simulink model "compDigital2"  (R2018a)
settings: Solver=VariableStepAuto  StartTime=0.0  StopTime=10.0  RelTol=1e-3
values from neighbouring files (symbols this model uses):
  Ts = 1/fs    (= 2e-05)    [transferencias_digitales.m]
undefined symbols (not defined in the file or in its folder): CtotalZ, Gtotalz, intZ
libraries: simulink x1
settings Model: Creator=Ignacio  LastModifiedBy=Ignacio

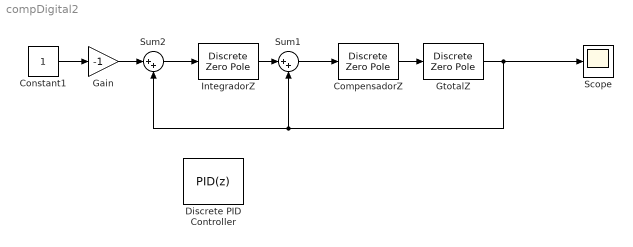
== system compDigital2 ==
  CompensadorZ : DiscreteZeroPole  Zeros=CtotalZ.Z{1,1}  Poles=CtotalZ.P{1,1}  Gain=CtotalZ.K  SampleTime=Ts
  Constant1 : Constant
  Discrete PID Controller : simulink/Continuous/PID Controller  Controller=PID  TimeDomain=Discrete-time  SampleTime=-1  IntegratorMethod=Forward Euler  FilterMethod=Forward Euler  Form=Parallel  UseFilter=on  ControllerParametersSource=internal  P=1  I=1  D=0  N=100  InitialConditionSource=internal  InitialConditionForIntegrator=0  InitialConditionForFilter=0  ExternalReset=none  LimitOutput=off  UpperSaturationLimit=inf  LowerSaturationLimit=-inf  LinearizeAsGain=off  AntiWindupMode=none  Kb=1  TrackingMode=off  Kt=1  PParamMin=[]  PParamMax=[]  IParamMin=[]  IParamMax=[]  DParamMin=[]  DParamMax=[]  NParamMin=[]  NParamMax=[]  KbParamMin=[]  KbParamMax=[]  KtParamMin=[]  KtParamMax=[]  POutMin=[]  POutMax=[]  IOutMin=[]  IOutMax=[]  DOutMin=[]  DOutMax=[]  NOutMin=[]  NOutMax=[]  KbOutMin=[]  KbOutMax=[]  KtOutMin=[]  KtOutMax=[]  IntegratorOutMin=[]  IntegratorOutMax=[]  FilterOutMin=[]  FilterOutMax=[]  SumOutMin=[]  SumOutMax=[]  SumI1OutMin=[]  SumI1OutMax=[]  SumI2OutMin=[]  SumI2OutMax=[]  SumI3OutMin=[]  SumI3OutMax=[]  SumDOutMin=[]  SumDOutMax=[]  SaturationOutMin=[]  SaturationOutMax=[]  IntegratorContinuousStateAttributes=''  IntegratorStateMustResolveToSignalObject=off  IntegratorRTWStateStorageClass=Auto  FilterContinuousStateAttributes=''  FilterStateMustResolveToSignalObject=off  FilterRTWStateStorageClass=Auto  DifferentiatorICPrevScaledInput=0  DifferentiatorOutMin=[]  DifferentiatorOutMax=[]  FilterDiffOutCoefMin=[]  FilterDiffOutCoefMax=[]  SumDenOutMin=[]  SumDenOutMax=[]  SumNumOutMin=[]  SumNumOutMax=[]  ReciprocalOutMin=[]  ReciprocalOutMax=[]  DivideOutMin=[]  DivideOutMax=[]  TunerSelectOption=Transfer Function Based (PID Tuner App)
  Gain : Gain  Gain=-1
  GtotalZ : DiscreteZeroPole  Zeros=Gtotalz.Z{1,1}  Poles=Gtotalz.P{1,1}  Gain=Gtotalz.K  SampleTime=Ts
  IntegradorZ : DiscreteZeroPole  Zeros=intZ.Z{1,1}  Poles=intZ.P{1,1}  Gain=intZ.K  SampleTime=Ts
  Scope : Scope
  Sum1 : Sum  Inputs=|++
  Sum2 : Sum  Inputs=|++
  wires:
  GtotalZ/1 -> Scope/1, Sum2/2, Sum1/2
  Sum1/1 -> CompensadorZ/1
  CompensadorZ/1 -> GtotalZ/1
  IntegradorZ/1 -> Sum1/1
  Sum2/1 -> IntegradorZ/1
  Constant1/1 -> Gain/1
  Gain/1 -> Sum2/1
